simulink model "test_stability_link_auto_speed_two_neurons_mod_switch"  (R2022a)
settings: Solver=VariableStepAuto  StartTime=0.0  StopTime=20  RelTol=1e-3
values from neighbouring files (symbols this model uses):
  Y = fft(theta)    [testStability.m]    (also in testStabilityTmp2.m)
undefined symbols (not defined in the file or in its folder): bar_amp, bar_amp_base, buff_amp, dfm, dfm_mod, dgsm_g, dsm, dsm_mod, dsp, dsp_mod, dsyn, dup, dup_mod, gfm, gfm_mod, gsm, gsm_mod, gsp, gsp_mod, gsyn, gup, gup_mod, Iapp, Iapp_mod, max_torque, noisePwr, rflx_g, sampleTime, sr_gain, switch_time, X, Z
libraries: sm_lib x6, simulink x4, nesl_utility x4
settings Model: Creator=chris  LastModifiedBy=chris

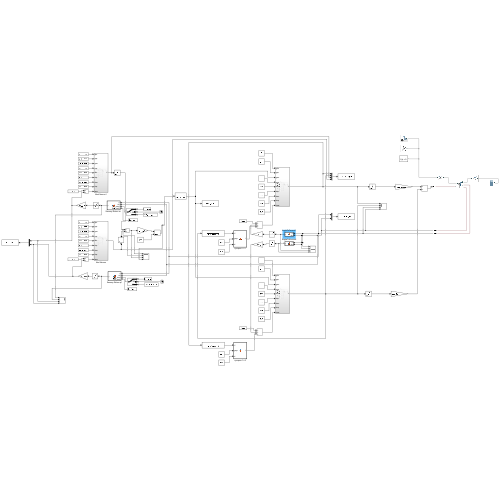
[thumbnail: Simulink's stored preview of the top-level diagram]
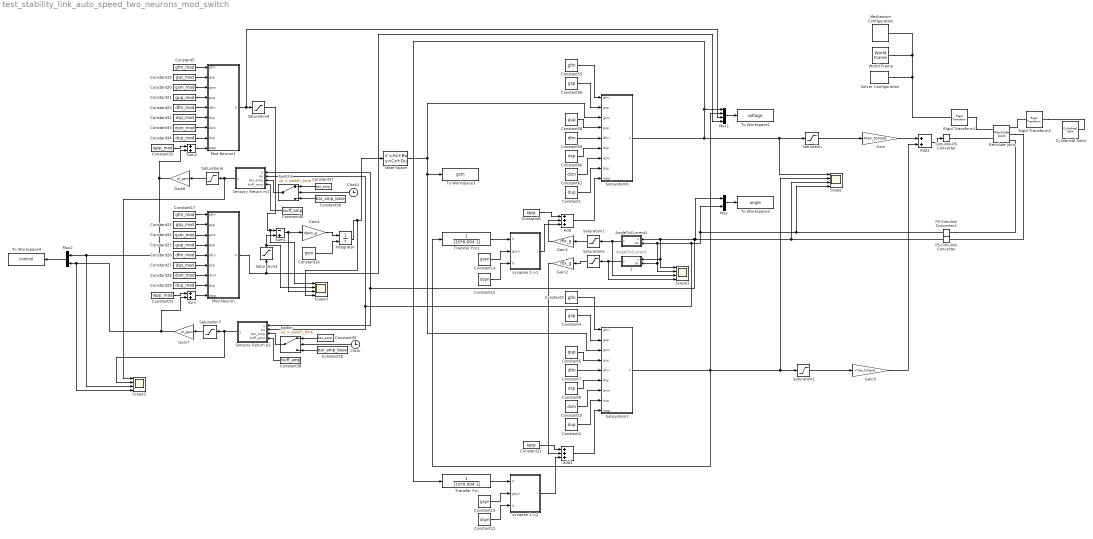
== system test_stability_link_auto_speed_two_neurons_mod_switch ==
  note: AngleToCurrent
  1 : MATLAB Function  TreatAsAtomicUnit=on
  Add : Sum  Inputs=+++
  Add1 : Sum  Inputs=+++
  Add2 : Sum
  AngleToCurrent1 : MATLAB Function  TreatAsAtomicUnit=on
  Clock : Clock
  Clock1 : Clock
  Constant1 : Constant  Value=dup
  Constant10 : Constant  Value=dsm
  Constant11 : Constant  Value=Iapp
  Constant12 : Constant  Value=dsyn
  Constant13 : Constant  Value=gsyn
  Constant14 : Constant  Value=gsyn
  Constant15 : Constant  Value=dsyn
  Constant16 : Constant  Value=gsm
  Constant17 : Constant  Value=gfm_mod
  Constant18 : Constant  Value=bar_amp_base
  Constant19 : Constant  Value=gsp_mod
  Constant2 : Constant  Value=dup
  Constant20 : Constant  Value=gsm_mod
  Constant21 : Constant  Value=gup_mod
  Constant22 : Constant  Value=dfm_mod
  Constant23 : Constant  Value=gsp_mod
  Constant24 : Constant  Value=gsm_mod
  Constant25 : Constant  Value=gup_mod
  Constant26 : Constant  Value=dfm_mod
  Constant27 : Constant  Value=dsp_mod
  Constant28 : Constant  Value=dsm_mod
  Constant29 : Constant  Value=dup_mod
  Constant3 : Constant  Value=gfm
  Constant30 : Constant  Value=bar_amp
  Constant31 : Constant  Value=Iapp_mod
  Constant32 : Constant  Value=dsp_mod
  Constant33 : Constant  Value=dsm_mod
  Constant34 : Constant  Value=dup_mod
  Constant35 : Constant  Value=Iapp_mod
  Constant36 : Constant  Value=bar_amp_base
  Constant37 : Constant  Value=bar_amp
  Constant38 : Constant  Value=buff_amp
  Constant4 : Constant  Value=gsp
  Constant40 : Constant  Value=buff_amp
  Constant5 : Constant  Value=gfm_mod
  Constant55 : Constant  Value=gfm
  Constant56 : Constant  Value=gsp
  Constant58 : Constant  Value=gup
  Constant59 : Constant  Value=dfm
  Constant6 : Constant  Value=gup
  Constant60 : Constant  Value=dsp
  Constant61 : Constant  Value=dsm
  Constant7 : Constant  Value=dfm
  Constant8 : Constant  Value=Iapp
  Constant9 : Constant  Value=dsp
  Cylindrical Solid : sm_lib/Body Elements/Cylindrical Solid  GraphicAmbientColor=[0.15 0.15 0.15 1.0]  BasedOnType=Density  CenterOfMass=[0 0 0]  CenterOfMassUnits=m  GraphicDiffuseColor=[0.5 0.5 0.5]  CylinderLength=0.5  CylinderLengthUnits=m  CylinderRadius=0.05  CylinderRadiusUnits=m  Density=1000  DensityUnits=kg/m^3  DoExposeReferenceFrame=on  GraphicEmissiveColor=[0.0 0.0 0.0 1.0]  ExportEntireGeometry=off  SerializedFrames=<Frames/>  MarkerShape=Sphere  MarkerSize=10  GraphicType=FromGeometry  InertiaType=CalculateFromGeometry  Mass=1  MassUnits=kg  MomentsOfInertia=[1 1 1]  MomentsOfInertiaUnits=kg*m^2  GraphicOpacity=1.0  ProductsOfInertia=[0 0 0]  ProductsOfInertiaUnits=kg*m^2  GraphicShininess=75  GraphicSpecularColor=[0.5 0.5 0.5 1.0]  GraphicVisPropType=SimpleVisualProperties
  Gain : Gain  Gain=max_torque
  Gain1 : Gain  Gain=rflx_g
  Gain2 : Gain  Gain=rflx_g
  Gain3 : Gain  Gain=-max_torque
  Gain4 : Gain  Gain=dgsm_g
  Gain6 : Gain  Gain=sr_gain
  Gain7 : Gain  Gain=sr_gain
  Integrator : Integrator  InitialConditionSource=external
  Mechanism Configuration : sm_lib/Utilities/Mechanism Configuration  UniformGravity=Constant  GravityVector=[0 0 -9.80665]  GravityUnits=m/s^2  LinearizationDelta=0.001  JointModeTransitionNonlinearIterations=2
  Mod Neuron : Subsystem
  Mod Neuron1 : Subsystem
  Mux : Mux  Inputs=2
  Mux1 : Mux
  Mux2 : Mux  Inputs=2
  PS-Simulink Converter : nesl_utility/PS-Simulink Converter  PhysicalDomain=network_engine_domain  SubClassName=ps_output  LeftPortType=input  RightPortType=output  PseudoPeriodic=off  Frequencies=[]  VectorFormat=inherit  Unit=inherit  AffineConversion=off
      settings: SourceProductBaseCode=SS,PW,VE
  PS-Simulink Converter1 : nesl_utility/PS-Simulink Converter  PhysicalDomain=network_engine_domain  SubClassName=ps_output  LeftPortType=input  RightPortType=output  PseudoPeriodic=off  Frequencies=[]  VectorFormat=inherit  Unit=inherit  AffineConversion=off
      settings: SourceProductBaseCode=SS,PW,VE
  Revolute Joint : sm_lib/Joints/Revolute Joint  JointMode=Normal  SenseConstraintForce=off  SenseConstraintForceX=off  SenseConstraintForceY=off  SenseConstraintForceZ=off  SenseConstraintTorque=off  SenseConstraintTorqueX=off  SenseConstraintTorqueY=off  SenseConstraintTorqueZ=off  SenseTotalForce=off  SenseTotalForceX=off  SenseTotalForceY=off  SenseTotalForceZ=off  SenseTotalTorque=off  SenseTotalTorqueX=off  SenseTotalTorqueY=off  SenseTotalTorqueZ=off  CompositeWrenchDir=FollowerOnBase  CompositeWrenchFrame=BaseFrame  EquilibriumPosition=0  EquilibriumPositionUnits=deg  SpringStiffness=0.0  SpringStiffnessUnits=N*m/deg  DampingCoefficient=0.01  DampingCoefficientUnits=N*m/(deg/s)  TorqueActuationMode=InputTorque  MotionActuationMode=ComputedMotion  SensePosition=on  SenseVelocity=on  SenseAcceleration=off  SenseTorqueForce=off  SenseLowerLimitTorqueForce=off  SenseUpperLimitTorqueForce=off  LowerLimitSpecify=off  LowerLimitBound=-90  LowerLimitBoundUnits=deg  LowerLimitStiffness=1e4  LowerLimitStiffnessUnits=N*m/deg  LowerLimitDamping=10  LowerLimitDampingUnits=N*m/(deg/s)  LowerLimitTransitionRegionWidth=0.1  LowerLimitTransitionRegionWidthUnits=deg  UpperLimitSpecify=off  UpperLimitBound=90  UpperLimitBoundUnits=deg  UpperLimitStiffness=1e4  UpperLimitStiffnessUnits=N*m/deg  UpperLimitDamping=10  UpperLimitDampingUnits=N*m/(deg/s)  UpperLimitTransitionRegionWidth=0.1  UpperLimitTransitionRegionWidthUnits=deg  PositionTargetSpecify=on  PositionTargetPriority=High  PositionTargetValue=20  PositionTargetValueUnits=deg  VelocityTargetSpecify=off  VelocityTargetPriority=High  VelocityTargetValue=0  VelocityTargetValueUnits=deg/s
  Rigid Transform1 : sm_lib/Frames and Transforms/Rigid Transform  TranslationMethod=None  TranslationStandardOffset=0.25  TranslationLengthUnit=m  TranslationStandardAxis=+X  TranslationCartesianOffset=[0 0 0]  TranslationROffset=0  TranslationROffsetUnits=m  TranslationZOffset=0  TranslationZOffsetUnits=m  TranslationThetaOffset=0  TranslationThetaOffsetUnits=deg  RotationMethod=RotationSequence  RotationAngleUnits=deg  RotationStandardAxis=+Y  RotationAngle=90  RotationArbitraryAxis=[0 0 1]  FollAlignAxisA=+X  BaseAlignAxisA=+Y  FollAlignAxisB=+Y  BaseAlignAxisB=+Z  RotationSequenceAxes=FollowerAxes  RotationSequence=XYX  RotationSequenceAngles=[0 90 90]  RotationSequenceAnglesUnits=deg  RotationMatrix=[1 0 0; 0 1 0; 0 0 1]
  Rigid Transform2 : sm_lib/Frames and Transforms/Rigid Transform  TranslationMethod=StandardAxis  TranslationStandardOffset=.25  TranslationLengthUnit=m  TranslationStandardAxis=+X  TranslationCartesianOffset=[0 0 0]  TranslationROffset=0  TranslationROffsetUnits=m  TranslationZOffset=0  TranslationZOffsetUnits=m  TranslationThetaOffset=0  TranslationThetaOffsetUnits=deg  RotationMethod=RotationSequence  RotationAngleUnits=deg  RotationStandardAxis=+Z  RotationAngle=90  RotationArbitraryAxis=[0 0 1]  FollAlignAxisA=+X  BaseAlignAxisA=+Y  FollAlignAxisB=+Y  BaseAlignAxisB=+Z  RotationSequenceAxes=FollowerAxes  RotationSequence=XYX  RotationSequenceAngles=[0 90 0]  RotationSequenceAnglesUnits=deg  RotationMatrix=[1 0 0; 0 1 0; 0 0 1]
  Saturation{,1..7} (8 alike) : Saturate  UpperLimit=1.0  LowerLimit=0.0
  Scope{,1..3} (4 alike) : Scope  NumInputPorts=4
  Sensory Return m1 : MATLAB Function  TreatAsAtomicUnit=on
  Sensory Return p1 : MATLAB Function  TreatAsAtomicUnit=on
  Simulink-PS Converter : nesl_utility/Simulink-PS Converter  PhysicalDomain=network_engine_domain  SubClassName=ps_input  LeftPortType=input  RightPortType=output  PseudoPeriodic=off  Frequencies=[]  NoiseDistribution=none  NoiseParameters=[]  Unit=1  AffineConversion=off  FilteringAndDerivatives=provide  SimscapeFilterOrder=1  InputFilterTimeConstant=0.001  UdotUserProvided=0
      settings: SourceProductBaseCode=SS,PW,VE
  Solver Configuration : nesl_utility/Solver Configuration  PhysicalDomain=network_engine_domain  SubClassName=solver  LeftPortType=input  RightPortType=generic  Tones=[]  Harmonics=[]  SimulateNoise=off  Profile=off  UseLocalSampling=off  EnableSwitchedLinearOptims=on  FrequencyDomain=off  UseCCode=off  RelTol=0.001  AbsTol=1e-06  MinStep=1e-09  ToWorkspace=off  RevertToSquareIcSolve=off  NumHomotopyIterations=100  PhasorMode=off  PhasorModeNumHarmonics=1  IndexReductionMethod=DerivativeReplacement  DoDC=off  ResidualTolerance=1e-09  UseLocalSolver=off  LocalSolverChoice=NE_BACKWARD_EULER_ADVANCER  LocalSolverSampleTime=0.001  DoFixedCost=off  MaxNonlinIter=3  MaxModeIter=2  ComputeImpulses=off  ImpulseIterations=2  LinearAlgebra=auto  LinearAlgebraNumThread=0  EquationFormulation=NE_TIME_EF  DelaysMemoryBudget=1024  AutomaticFiltering=on  FilteringTimeConstant=0.001  PartitionStorageMethod=AS_NEEDED  PartitionMemoryBudget=1024  PartitionMethod=ROBUST
      settings: SourceProductBaseCode=SS,PW,VE
  State-Space : StateSpace  A=-10  B=10  D=0  InitialCondition=gsm
  Subsystem1 : Subsystem
  Subsystem6 : Subsystem
  Sum : Sum
  Sum1 : Sum  Inputs=-+
  Sum2 : Sum
  Switch : Switch  Criteria=u2 > Threshold  Threshold=switch_time  SaturateOnIntegerOverflow=off  InputSameDT=off
  Switch1 : Switch  Criteria=u2 > Threshold  Threshold=switch_time  SaturateOnIntegerOverflow=off  InputSameDT=off
  To Workspace1 : ToWorkspace  VariableName=voltage  SaveFormat=Structure With Time  SampleTime=sampleTime
  To Workspace2 : ToWorkspace  VariableName=angle  SaveFormat=Structure With Time  SampleTime=sampleTime
  To Workspace3 : ToWorkspace  VariableName=gsm  SaveFormat=Structure With Time  SampleTime=sampleTime
  To Workspace4 : ToWorkspace  VariableName=control  SaveFormat=Structure With Time  SampleTime=sampleTime
  Transfer Fcn : TransferFcn  Denominator=[10*0.004 1]
  Transfer Fcn1 : TransferFcn  Denominator=[10*0.004 1]
  World Frame : sm_lib/Frames and Transforms/World Frame
  synapse 1->1 : MATLAB Function  TreatAsAtomicUnit=on
  synapse 1->2 : MATLAB Function  TreatAsAtomicUnit=on
  wires:
  Subsystem6/1(V) -> Transfer Fcn/1, Mux1/1, Scope/1, Saturation/1
  Constant60/1 -> Subsystem6/6(dsp)
  Constant1/1 -> Subsystem6/8(dup)
  Constant59/1 -> Subsystem6/5(dfm)
  Constant61/1 -> Subsystem6/7(dsm)
  Constant56/1 -> Subsystem6/2(gsp)
  Constant58/1 -> Subsystem6/4(gup)
  Constant55/1 -> Subsystem6/1(gfm)
  Saturation/1 -> Gain/1
  Add/1 -> Subsystem6/9(Iapp)
  Constant8/1 -> Add/1
  Mux/1 -> To Workspace2/1
  PS-Simulink Converter1/1 -> Scope/4, Mux/2, Scope1/2, 1/2(du), AngleToCurrent1/2(du), Sensory Return m1/2(du), Sensory Return p1/2(du)
  Gain1/1 -> Add/2
  Constant9/1 -> Subsystem1/6(dsp)
  Constant11/1 -> Add1/1
  Constant10/1 -> Subsystem1/7(dsm)
  Constant3/1 -> Subsystem1/1(gfm)
  Constant4/1 -> Subsystem1/2(gsp)
  Constant7/1 -> Subsystem1/5(dfm)
  Add1/1 -> Subsystem1/9(Iapp)
  Constant6/1 -> Subsystem1/4(gup)
  Constant2/1 -> Subsystem1/8(dup)
  Gain2/1 -> Add1/2
  Subsystem1/1(V) -> Transfer Fcn1/1, Saturation2/1, Scope/2, Mux1/2
  Saturation2/1 -> Gain3/1
  Add2/1 -> Simulink-PS Converter/1
  Gain/1 -> Add2/1
  Gain3/1 -> Add2/2
  synapse 1->2/1(I) -> Add1/3
  synapse 1->1/1(I) -> Add/3
  Transfer Fcn/1 -> synapse 1->2/1(V)
  Transfer Fcn1/1 -> synapse 1->1/1(V)
  Constant13/1 -> synapse 1->2/2(gsyn)
  Constant12/1 -> synapse 1->2/3(d)
  Constant15/1 -> synapse 1->1/3(d)
  Constant14/1 -> synapse 1->1/2(gsyn)
  Mux1/1 -> To Workspace1/1
  Sum/1 -> Mod Neuron/9(Iapp)
  Constant17/1 -> Mod Neuron/1(gfm)
  Constant23/1 -> Mod Neuron/2(gsp)
  Constant31/1 -> Sum/1
  Constant28/1 -> Mod Neuron/7(dsm)
  Constant26/1 -> Mod Neuron/5(dfm)
  Constant27/1 -> Mod Neuron/6(dsp)
  Constant24/1 -> Mod Neuron/3(gsm)
  Constant25/1 -> Mod Neuron/4(gup)
  Constant29/1 -> Mod Neuron/8(dup)
  PS-Simulink Converter/1 -> Scope/3, Scope1/1, 1/1(u), AngleToCurrent1/1(u), Sensory Return m1/1(u), Sensory Return p1/1(u), Mux/1
  Constant16/1 -> Integrator/2
  Mod Neuron/1(V) -> Saturation3/1, Mux1/4
  Saturation4/1 -> Scope3/1, Sum1/1
  Saturation3/1 -> Scope3/2, Sum1/2
  Integrator/1 -> State-Space/1, Scope3/4
  State-Space/1 -> Subsystem1/3(gsm), To Workspace3/1, Subsystem6/3(gsm)
  Gain4/1 -> Integrator/1
  Sum1/1 -> Scope3/3, Gain4/1
  Sum2/1 -> Mod Neuron1/9(Iapp)
  Constant22/1 -> Mod Neuron1/5(dfm)
  Constant35/1 -> Sum2/1
  Constant21/1 -> Mod Neuron1/4(gup)
  Constant32/1 -> Mod Neuron1/6(dsp)
  Constant20/1 -> Mod Neuron1/3(gsm)
  Constant33/1 -> Mod Neuron1/7(dsm)
  Constant5/1 -> Mod Neuron1/1(gfm)
  Constant19/1 -> Mod Neuron1/2(gsp)
  Constant34/1 -> Mod Neuron1/8(dup)
  Sensory Return m1/1(y) -> Scope2/1, Saturation6/1
  Mod Neuron1/1(V) -> Mux1/3, Saturation4/1
  Mux2/1 -> To Workspace4/1
  Saturation1/1 -> Gain1/1
  Saturation5/1 -> Gain2/1
  Gain6/1 -> Scope2/3, Mux2/1, Sum2/2
  Sensory Return p1/1(y) -> Scope2/2, Saturation7/1
  Gain7/1 -> Sum/2, Mux2/2, Scope2/4
  AngleToCurrent1/1(y) -> Saturation1/1, Scope1/3
  1/1(y) -> Scope1/4, Saturation5/1
  Saturation6/1 -> Gain6/1
  Saturation7/1 -> Gain7/1
  Constant30/1 -> Switch/1
  Clock/1 -> Switch/2
  Constant18/1 -> Switch/3
  Switch/1 -> Sensory Return p1/3(bar_amp)
  Switch1/1 -> Sensory Return m1/3(bar_amp)
  Constant37/1 -> Switch1/1
  Clock1/1 -> Switch1/2
  Constant36/1 -> Switch1/3
  Constant38/1 -> Sensory Return p1/4(buff_amp)
  Constant40/1 -> Sensory Return m1/4(buff_amp)
  connections:
  Solver Configuration/RConn1 -- Mechanism Configuration/RConn1 -- World Frame/RConn1 -- Rigid Transform1/LConn1
  Rigid Transform1/RConn1 -- Revolute Joint/LConn1
  Simulink-PS Converter/RConn1 -- Revolute Joint/LConn2
  Rigid Transform2/RConn1 -- Cylindrical Solid/RConn1
  Rigid Transform2/LConn1 -- Revolute Joint/RConn1
  Revolute Joint/RConn2 -- PS-Simulink Converter/LConn1
  PS-Simulink Converter1/LConn1 -- Revolute Joint/RConn3

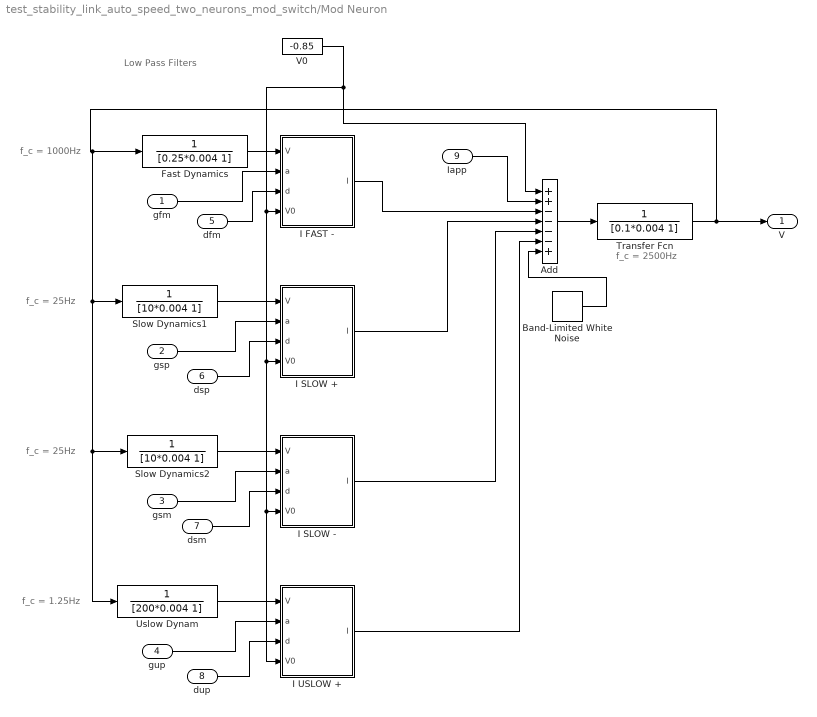
== system test_stability_link_auto_speed_two_neurons_mod_switch/Mod Neuron ==
  note: f_c = 2500Hz
  note: f_c = 1.25Hz
  note: f_c = 25Hz
  note: f_c = 1000Hz
  note: Low Pass Filters
  note: f_c = 25Hz
  gfm : Inport
  gsp : Inport  Port=2
  gsm : Inport  Port=3
  gup : Inport  Port=4
  dfm : Inport  Port=5
  dsp : Inport  Port=6
  dsm : Inport  Port=7
  dup : Inport  Port=8
  Iapp : Inport  Port=9
  Add : Sum  Inputs=++----+
  Band-Limited White Noise : simulink/Sources/Band-Limited White Noise  Cov=[0.0]  Ts=0.1  seed=[23341]
  Fast Dynamics : TransferFcn  Denominator=[0.25*0.004 1]
  I FAST - : MATLAB Function  TreatAsAtomicUnit=on
  I SLOW + : MATLAB Function  TreatAsAtomicUnit=on
  I SLOW - : MATLAB Function  TreatAsAtomicUnit=on
  I USLOW + : MATLAB Function  TreatAsAtomicUnit=on
  Slow Dynamics1 : TransferFcn  Denominator=[10*0.004 1]
  Slow Dynamics2 : TransferFcn  Denominator=[10*0.004 1]
  Transfer Fcn : TransferFcn  Denominator=[0.1*0.004 1]
  Uslow Dynam : TransferFcn  Denominator=[200*0.004 1]
  V0 : Constant  Value=-0.85
  V : Outport
  wires:
  dup/1 -> I USLOW +/3(d)
  gsm/1 -> I SLOW -/2(a)
  dsm/1 -> I SLOW -/3(d)
  gup/1 -> I USLOW +/2(a)
  Iapp/1 -> Add/2
  Uslow Dynam/1 -> I USLOW +/1(V)
  Add/1 -> Transfer Fcn/1
  Slow Dynamics1/1 -> I SLOW +/1(V)
  Slow Dynamics2/1 -> I SLOW -/1(V)
  I FAST -/1(I) -> Add/3
  I USLOW +/1(I) -> Add/6
  V0/1 -> I USLOW +/4(V0), I SLOW -/4(V0), I SLOW +/4(V0), I FAST -/4(V0), Add/1
  dsp/1 -> I SLOW +/3(d)
  gsp/1 -> I SLOW +/2(a)
  dfm/1 -> I FAST -/3(d)
  gfm/1 -> I FAST -/2(a)
  Fast Dynamics/1 -> I FAST -/1(V)
  I SLOW -/1(I) -> Add/5
  Transfer Fcn/1 -> V/1, Uslow Dynam/1, Slow Dynamics2/1, Slow Dynamics1/1, Fast Dynamics/1
  I SLOW +/1(I) -> Add/4
  Band-Limited White Noise/1 -> Add/7

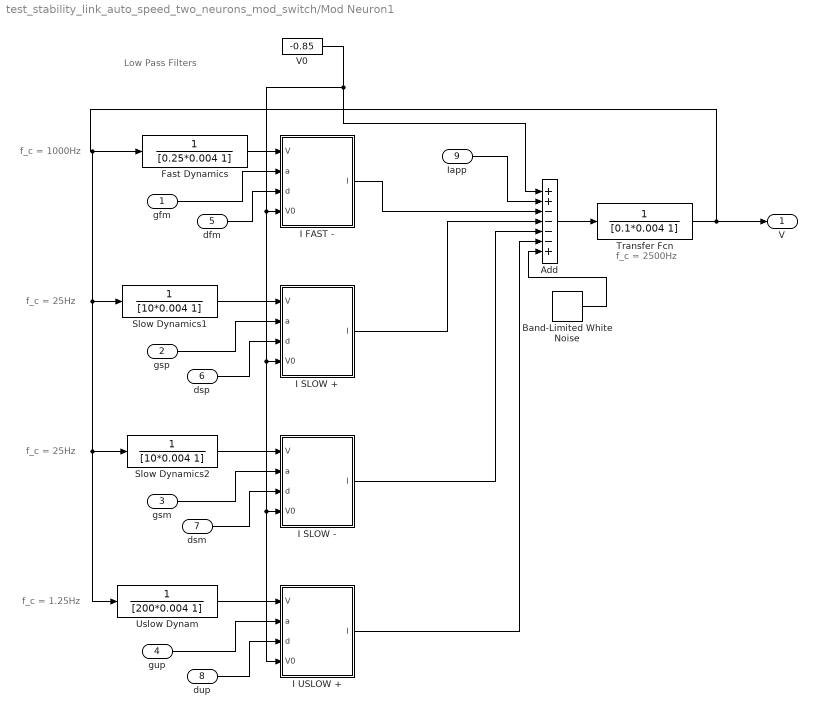
== system test_stability_link_auto_speed_two_neurons_mod_switch/Mod Neuron1 ==
  note: f_c = 2500Hz
  note: f_c = 1.25Hz
  note: f_c = 25Hz
  note: f_c = 1000Hz
  note: Low Pass Filters
  note: f_c = 25Hz
  gfm : Inport
  gsp : Inport  Port=2
  gsm : Inport  Port=3
  gup : Inport  Port=4
  dfm : Inport  Port=5
  dsp : Inport  Port=6
  dsm : Inport  Port=7
  dup : Inport  Port=8
  Iapp : Inport  Port=9
  Add : Sum  Inputs=++----+
  Band-Limited White Noise : simulink/Sources/Band-Limited White Noise  Cov=[0.0]  Ts=0.1  seed=[23341]
  Fast Dynamics : TransferFcn  Denominator=[0.25*0.004 1]
  I FAST - : MATLAB Function  TreatAsAtomicUnit=on
  I SLOW + : MATLAB Function  TreatAsAtomicUnit=on
  I SLOW - : MATLAB Function  TreatAsAtomicUnit=on
  I USLOW + : MATLAB Function  TreatAsAtomicUnit=on
  Slow Dynamics1 : TransferFcn  Denominator=[10*0.004 1]
  Slow Dynamics2 : TransferFcn  Denominator=[10*0.004 1]
  Transfer Fcn : TransferFcn  Denominator=[0.1*0.004 1]
  Uslow Dynam : TransferFcn  Denominator=[200*0.004 1]
  V0 : Constant  Value=-0.85
  V : Outport
  wires:
  dup/1 -> I USLOW +/3(d)
  gsm/1 -> I SLOW -/2(a)
  dsm/1 -> I SLOW -/3(d)
  gup/1 -> I USLOW +/2(a)
  Iapp/1 -> Add/2
  Uslow Dynam/1 -> I USLOW +/1(V)
  Add/1 -> Transfer Fcn/1
  Slow Dynamics1/1 -> I SLOW +/1(V)
  Slow Dynamics2/1 -> I SLOW -/1(V)
  I FAST -/1(I) -> Add/3
  I USLOW +/1(I) -> Add/6
  V0/1 -> I USLOW +/4(V0), I SLOW -/4(V0), I SLOW +/4(V0), I FAST -/4(V0), Add/1
  dsp/1 -> I SLOW +/3(d)
  gsp/1 -> I SLOW +/2(a)
  dfm/1 -> I FAST -/3(d)
  gfm/1 -> I FAST -/2(a)
  Fast Dynamics/1 -> I FAST -/1(V)
  I SLOW -/1(I) -> Add/5
  Transfer Fcn/1 -> V/1, Uslow Dynam/1, Slow Dynamics2/1, Slow Dynamics1/1, Fast Dynamics/1
  I SLOW +/1(I) -> Add/4
  Band-Limited White Noise/1 -> Add/7

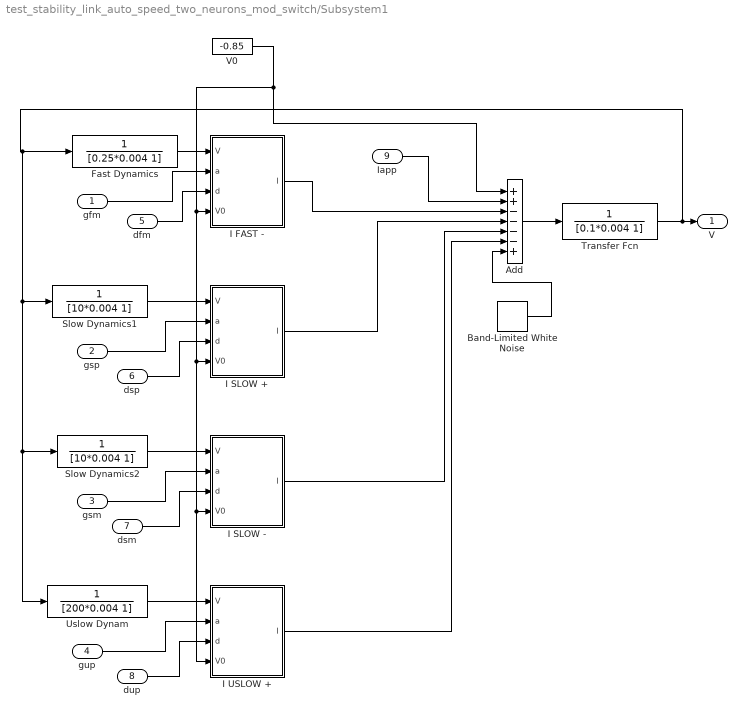
== system test_stability_link_auto_speed_two_neurons_mod_switch/Subsystem1 ==
  gfm : Inport
  gsp : Inport  Port=2
  gsm : Inport  Port=3
  gup : Inport  Port=4
  dfm : Inport  Port=5
  dsp : Inport  Port=6
  dsm : Inport  Port=7
  dup : Inport  Port=8
  Iapp : Inport  Port=9
  Add : Sum  Inputs=++----+
  Band-Limited White Noise : simulink/Sources/Band-Limited White Noise  Cov=[noisePwr]  Ts=0.001  seed=floor(rand(1)*250000)
  Fast Dynamics : TransferFcn  Denominator=[0.25*0.004 1]
  I FAST - : MATLAB Function  TreatAsAtomicUnit=on
  I SLOW + : MATLAB Function  TreatAsAtomicUnit=on
  I SLOW - : MATLAB Function  TreatAsAtomicUnit=on
  I USLOW + : MATLAB Function  TreatAsAtomicUnit=on
  Slow Dynamics1 : TransferFcn  Denominator=[10*0.004 1]
  Slow Dynamics2 : TransferFcn  Denominator=[10*0.004 1]
  Transfer Fcn : TransferFcn  Denominator=[0.1*0.004 1]
  Uslow Dynam : TransferFcn  Denominator=[200*0.004 1]
  V0 : Constant  Value=-0.85
  V : Outport
  wires:
  dup/1 -> I USLOW +/3(d)
  gsm/1 -> I SLOW -/2(a)
  dsm/1 -> I SLOW -/3(d)
  gup/1 -> I USLOW +/2(a)
  Iapp/1 -> Add/2
  Uslow Dynam/1 -> I USLOW +/1(V)
  Add/1 -> Transfer Fcn/1
  Slow Dynamics1/1 -> I SLOW +/1(V)
  Slow Dynamics2/1 -> I SLOW -/1(V)
  I FAST -/1(I) -> Add/3
  I USLOW +/1(I) -> Add/6
  V0/1 -> I USLOW +/4(V0), I SLOW -/4(V0), I SLOW +/4(V0), I FAST -/4(V0), Add/1
  dsp/1 -> I SLOW +/3(d)
  gsp/1 -> I SLOW +/2(a)
  dfm/1 -> I FAST -/3(d)
  gfm/1 -> I FAST -/2(a)
  Fast Dynamics/1 -> I FAST -/1(V)
  I SLOW -/1(I) -> Add/5
  Transfer Fcn/1 -> Uslow Dynam/1, Slow Dynamics2/1, Slow Dynamics1/1, Fast Dynamics/1, V/1
  I SLOW +/1(I) -> Add/4
  Band-Limited White Noise/1 -> Add/7

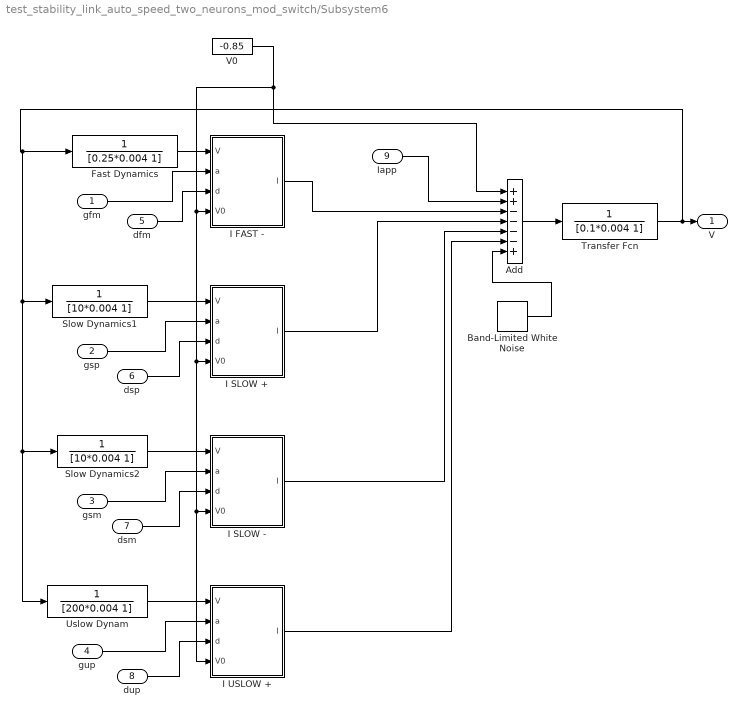
== system test_stability_link_auto_speed_two_neurons_mod_switch/Subsystem6 ==
  gfm : Inport
  gsp : Inport  Port=2
  gsm : Inport  Port=3
  gup : Inport  Port=4
  dfm : Inport  Port=5
  dsp : Inport  Port=6
  dsm : Inport  Port=7
  dup : Inport  Port=8
  Iapp : Inport  Port=9
  Add : Sum  Inputs=++----+
  Band-Limited White Noise : simulink/Sources/Band-Limited White Noise  Cov=[noisePwr]  Ts=0.001  seed=floor(rand(1)*250000)
  Fast Dynamics : TransferFcn  Denominator=[0.25*0.004 1]
  I FAST - : MATLAB Function  TreatAsAtomicUnit=on
  I SLOW + : MATLAB Function  TreatAsAtomicUnit=on
  I SLOW - : MATLAB Function  TreatAsAtomicUnit=on
  I USLOW + : MATLAB Function  TreatAsAtomicUnit=on
  Slow Dynamics1 : TransferFcn  Denominator=[10*0.004 1]
  Slow Dynamics2 : TransferFcn  Denominator=[10*0.004 1]
  Transfer Fcn : TransferFcn  Denominator=[0.1*0.004 1]
  Uslow Dynam : TransferFcn  Denominator=[200*0.004 1]
  V0 : Constant  Value=-0.85
  V : Outport
  wires:
  dup/1 -> I USLOW +/3(d)
  gsm/1 -> I SLOW -/2(a)
  dsm/1 -> I SLOW -/3(d)
  gup/1 -> I USLOW +/2(a)
  Iapp/1 -> Add/2
  Uslow Dynam/1 -> I USLOW +/1(V)
  Add/1 -> Transfer Fcn/1
  Slow Dynamics1/1 -> I SLOW +/1(V)
  Slow Dynamics2/1 -> I SLOW -/1(V)
  I FAST -/1(I) -> Add/3
  I USLOW +/1(I) -> Add/6
  V0/1 -> I USLOW +/4(V0), I SLOW -/4(V0), I SLOW +/4(V0), I FAST -/4(V0), Add/1
  dsp/1 -> I SLOW +/3(d)
  gsp/1 -> I SLOW +/2(a)
  dfm/1 -> I FAST -/3(d)
  gfm/1 -> I FAST -/2(a)
  Fast Dynamics/1 -> I FAST -/1(V)
  I SLOW -/1(I) -> Add/5
  Transfer Fcn/1 -> Uslow Dynam/1, Slow Dynamics2/1, Slow Dynamics1/1, Fast Dynamics/1, V/1
  I SLOW +/1(I) -> Add/4
  Band-Limited White Noise/1 -> Add/7

== matlab function test_stability_link_auto_speed_two_neurons_mod_switch/Subsystem1/I FAST - ==
  data: V input; I output; a input; d input; V0 input
function I = fcn(V,a,d,V0)

I = a*(tanh(V-d)-tanh(V0-d));

== matlab function test_stability_link_auto_speed_two_neurons_mod_switch/Sensory Return p1 ==
  data: u input; du input; y output; bar_amp input; buff_amp input
function y = fcn(u, du, bar_amp, buff_amp)

yu = tanh( 40*(abs(wrapToPi(u)) - abs(wrapToPi(bar_amp)) - buff_amp) );
ydu = (tanh(20*(du+0.1)) - tanh(20*(du-0.1)))/2 - 1;
y = yu + ydu;

== matlab function test_stability_link_auto_speed_two_neurons_mod_switch/Mod Neuron1/I USLOW + ==
  data: V input; I output; a input; d input; V0 input
function I = fcn(V,a,d,V0)

I = a*(tanh(V-d)-tanh(V0-d));

== matlab function test_stability_link_auto_speed_two_neurons_mod_switch/synapse 1->2 ==
  data: V input; I output; gsyn input; d input
function I = fcn(V,gsyn,d)

I = gsyn*(tanh(2*(V-d))+1)/2;

== matlab function test_stability_link_auto_speed_two_neurons_mod_switch/Mod Neuron/I SLOW + ==
  data: V input; I output; a input; d input; V0 input
function I = fcn(V,a,d,V0)

I = a*(tanh(V-d)-tanh(V0-d));

== matlab function test_stability_link_auto_speed_two_neurons_mod_switch/Mod Neuron/I SLOW - ==
  data: V input; I output; a input; d input; V0 input
function I = fcn(V,a,d,V0)

I = a*(tanh(V-d)-tanh(V0-d));

== matlab function test_stability_link_auto_speed_two_neurons_mod_switch/Mod Neuron/I USLOW + ==
  data: V input; I output; a input; d input; V0 input
function I = fcn(V,a,d,V0)

I = a*(tanh(V-d)-tanh(V0-d));

== matlab function test_stability_link_auto_speed_two_neurons_mod_switch/Sensory Return m1 ==
  data: u input; du input; y output; bar_amp input; buff_amp input
function y = fcn(u, du, bar_amp, buff_amp)

yu = tanh( 40*(abs(wrapToPi(bar_amp)) - abs(wrapToPi(u)) - buff_amp) ) ;
ydu = (tanh(20*(du+0.1)) - tanh(20*(du-0.1)))/2 - 1;
y = yu + ydu;

== matlab function test_stability_link_auto_speed_two_neurons_mod_switch/AngleToCurrent1 ==
  data: u input; y output; du input
function y = fcn(u, du)
uy = (1-tanh(15*(sin(u)-0.05)))/2 - 1;
duy = (tanh(5*(du+0.5)) - tanh(5*(du-0.5)))/2;
y = uy + duy;

== matlab function test_stability_link_auto_speed_two_neurons_mod_switch/Subsystem6/I FAST - ==
  data: V input; I output; a input; d input; V0 input
function I = fcn(V,a,d,V0)

I = a*(tanh(V-d)-tanh(V0-d));

== matlab function test_stability_link_auto_speed_two_neurons_mod_switch/Subsystem6/I SLOW + ==
  data: V input; I output; a input; d input; V0 input
function I = fcn(V,a,d,V0)

I = a*(tanh(V-d)-tanh(V0-d));

== matlab function test_stability_link_auto_speed_two_neurons_mod_switch/Subsystem1/I SLOW + ==
  data: V input; I output; a input; d input; V0 input
function I = fcn(V,a,d,V0)

I = a*(tanh(V-d)-tanh(V0-d));

== matlab function test_stability_link_auto_speed_two_neurons_mod_switch/Subsystem6/I SLOW - ==
  data: V input; I output; a input; d input; V0 input
function I = fcn(V,a,d,V0)

I = a*(tanh(V-d)-tanh(V0-d));

== matlab function test_stability_link_auto_speed_two_neurons_mod_switch/Subsystem6/I USLOW + ==
  data: V input; I output; a input; d input; V0 input
function I = fcn(V,a,d,V0)

I = a*(tanh(V-d)-tanh(V0-d));

== matlab function test_stability_link_auto_speed_two_neurons_mod_switch/Subsystem1/I SLOW - ==
  data: V input; I output; a input; d input; V0 input
function I = fcn(V,a,d,V0)

I = a*(tanh(V-d)-tanh(V0-d));

== matlab function test_stability_link_auto_speed_two_neurons_mod_switch/Subsystem1/I USLOW + ==
  data: V input; I output; a input; d input; V0 input
function I = fcn(V,a,d,V0)

I = a*(tanh(V-d)-tanh(V0-d));

== matlab function test_stability_link_auto_speed_two_neurons_mod_switch/synapse 1->1 ==
  data: V input; I output; gsyn input; d input
function I = fcn(V,gsyn,d)

I = gsyn*(tanh(2*(V-d))+1)/2;

== matlab function test_stability_link_auto_speed_two_neurons_mod_switch/Mod Neuron/I FAST - ==
  data: V input; I output; a input; d input; V0 input
function I = fcn(V,a,d,V0)

I = a*(tanh(V-d)-tanh(V0-d));

== matlab function test_stability_link_auto_speed_two_neurons_mod_switch/1 ==
  data: u input; y output; du input
function y = fcn(u, du)
uy = (1+tanh(15*(sin(u)+0.05)))/2 - 1;
duy = (tanh(5*(du+0.5)) - tanh(5*(du-0.5)))/2;
y = uy + duy;

== matlab function test_stability_link_auto_speed_two_neurons_mod_switch/Mod Neuron1/I FAST - ==
  data: V input; I output; a input; d input; V0 input
function I = fcn(V,a,d,V0)

I = a*(tanh(V-d)-tanh(V0-d));

== matlab function test_stability_link_auto_speed_two_neurons_mod_switch/Mod Neuron1/I SLOW + ==
  data: V input; I output; a input; d input; V0 input
function I = fcn(V,a,d,V0)

I = a*(tanh(V-d)-tanh(V0-d));

== matlab function test_stability_link_auto_speed_two_neurons_mod_switch/Mod Neuron1/I SLOW - ==
  data: V input; I output; a input; d input; V0 input
function I = fcn(V,a,d,V0)

I = a*(tanh(V-d)-tanh(V0-d));
